simulink library "sixDoFDynamics_cl"  (R2020a)
settings: Solver=VariableStepAuto  StartTime=0.0  StopTime=10.0  RelTol=1e-3
undefined symbols (not defined in the file): init_B_vKite, init_Euler, init_OwB, init_rKite, invJKite, jKite, mKite
libraries: vrlib x2, sharedutil x1, makeOcB_cl x1
settings Model: Creator=Ayaz  LastModifiedBy=Ayaz

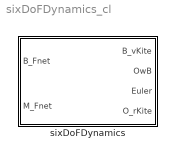
== system sixDoFDynamics_cl ==
  sixDoFDynamics : Subsystem

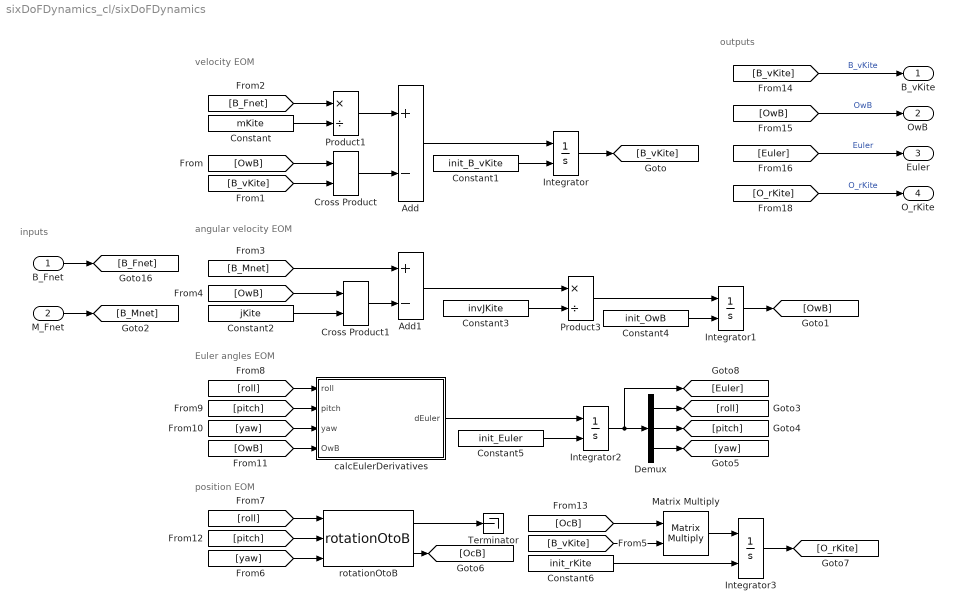
== system sixDoFDynamics_cl/sixDoFDynamics ==
  note: outputs
  note: inputs
  note: position EOM
  note: Euler angles EOM
  note: angular velocity EOM
  note: velocity EOM
  B_Fnet : Inport
  M_Fnet : Inport  Port=2
  Add : Sum  Inputs=+-
  Add1 : Sum  Inputs=+-
  Constant : Constant  Value=mKite
  Constant1 : Constant  Value=init_B_vKite
  Constant2 : Constant  Value=jKite
  Constant3 : Constant  Value=invJKite
  Constant4 : Constant  Value=init_OwB
  Constant5 : Constant  Value=init_Euler
  Constant6 : Constant  Value=init_rKite
  Cross Product : vrlib/Utilities/Cross Product
  Cross Product1 : vrlib/Utilities/Cross Product
  Demux : Demux  Outputs=3
  Integrator{,1..3} (4 alike) : Integrator  InitialConditionSource=external
  Matrix Multiply : Product  Multiplication=Matrix(*)
  Product1 : Product  Inputs=*/
  Product3 : Product  Inputs=*/
  Terminator : Terminator
  calcEulerDerivatives : Subsystem
  rotationOtoB : makeOcB_cl/rotationOtoB  SystemSampleTime=-1  Latency=0  AutoFrameSizeCalculation=off
  B_vKite : Outport
  OwB : Outport  Port=2
  Euler : Outport  Port=3
  O_rKite : Outport  Port=4
  wires:
  [OwB] -> Cross Product/1
  [B_vKite] -> Cross Product/2
  B_Fnet/1 -> [B_Fnet]
  [B_Fnet] -> Product1/1
  Constant/1 -> Product1/2
  Cross Product/1 -> Add/2
  Product1/1 -> Add/1
  Add/1 -> Integrator/1
  Constant1/1 -> Integrator/2
  Integrator/1 -> [B_vKite]
  M_Fnet/1 -> [B_Mnet]
  [OwB] -> Cross Product1/1
  Constant2/1 -> Cross Product1/2
  Cross Product1/1 -> Add1/2
  [B_Mnet] -> Add1/1
  Add1/1 -> Product3/1
  Constant3/1 -> Product3/2
  Product3/1 -> Integrator1/1
  Constant4/1 -> Integrator1/2
  Integrator1/1 -> [OwB]
  [roll] -> calcEulerDerivatives/1(roll)
  [pitch] -> calcEulerDerivatives/2(pitch)
  [yaw] -> calcEulerDerivatives/3(yaw)
  [OwB] -> calcEulerDerivatives/4(OwB)
  calcEulerDerivatives/1(dEuler) -> Integrator2/1
  Constant5/1 -> Integrator2/2
  Demux/1 -> [roll]
  Demux/2 -> [pitch]
  Demux/3 -> [yaw]
  Integrator2/1 -> [Euler], Demux/1
  [pitch] -> rotationOtoB/2
  [roll] -> rotationOtoB/1
  [yaw] -> rotationOtoB/3
  rotationOtoB/2 -> [OcB]
  [B_vKite] -> Matrix Multiply/2
  [OcB] -> Matrix Multiply/1
  rotationOtoB/1 -> Terminator/1
  Matrix Multiply/1 -> Integrator3/1
  Constant6/1 -> Integrator3/2
  Integrator3/1 -> [O_rKite]
  [B_vKite] -> B_vKite/1  "B_vKite"
  [OwB] -> OwB/1  "OwB"
  [Euler] -> Euler/1  "Euler"
  [O_rKite] -> O_rKite/1  "O_rKite"

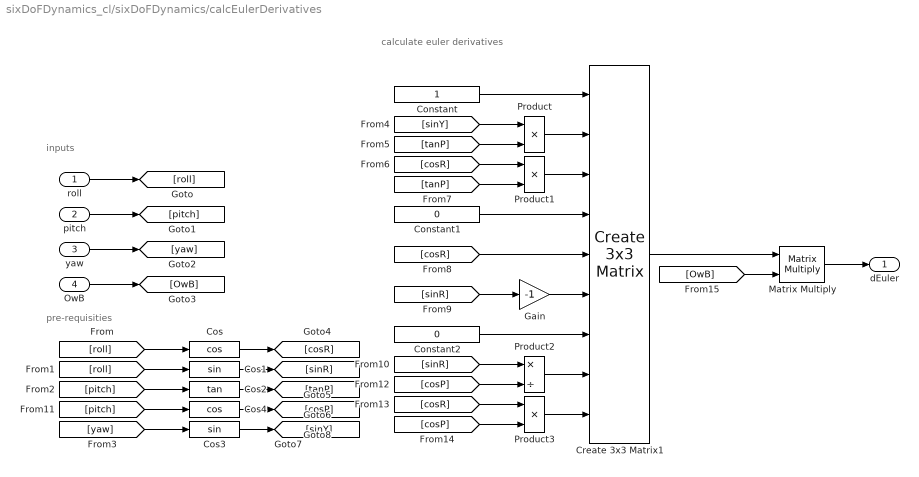
== system sixDoFDynamics_cl/sixDoFDynamics/calcEulerDerivatives ==
  note: calculate euler derivatives
  note: pre-requisities
  note: inputs
  roll : Inport
  pitch : Inport  Port=2
  yaw : Inport  Port=3
  OwB : Inport  Port=4
  Constant : Constant
  Constant1 : Constant  Value=0
  Constant2 : Constant  Value=0
  Cos : Trigonometry  Operator=cos
  Cos1 : Trigonometry
  Cos2 : Trigonometry  Operator=tan
  Cos3 : Trigonometry
  Cos4 : Trigonometry  Operator=cos
  Create 3x3 Matrix1 : sharedutil/Create 3x3 Matrix  aMode=aMode
      settings: SourceProductBaseCode=AE,PW,MT,VE,VP
  Gain : Gain  Gain=-1
  Matrix Multiply : Product  Multiplication=Matrix(*)
  Product : Product
  Product1 : Product
  Product2 : Product  Inputs=*/
  Product3 : Product
  dEuler : Outport
  wires:
  roll/1 -> [roll]
  pitch/1 -> [pitch]
  yaw/1 -> [yaw]
  OwB/1 -> [OwB]
  [roll] -> Cos/1
  [roll] -> Cos1/1
  [pitch] -> Cos2/1
  [yaw] -> Cos3/1
  Cos/1 -> [cosR]
  Cos1/1 -> [sinR]
  Cos2/1 -> [tanP]
  Cos3/1 -> [sinY]
  Constant/1 -> Create 3x3 Matrix1/1
  Product/1 -> Create 3x3 Matrix1/2
  [sinY] -> Product/1
  [tanP] -> Product/2
  Product1/1 -> Create 3x3 Matrix1/3
  [cosR] -> Product1/1
  [tanP] -> Product1/2
  Constant1/1 -> Create 3x3 Matrix1/4
  [cosR] -> Create 3x3 Matrix1/5
  [sinR] -> Gain/1
  Gain/1 -> Create 3x3 Matrix1/6
  Constant2/1 -> Create 3x3 Matrix1/7
  Product3/1 -> Create 3x3 Matrix1/9
  Product2/1 -> Create 3x3 Matrix1/8
  [sinR] -> Product2/1
  Cos4/1 -> [cosP]
  [pitch] -> Cos4/1
  [cosP] -> Product2/2
  [cosR] -> Product3/1
  [cosP] -> Product3/2
  Create 3x3 Matrix1/1 -> Matrix Multiply/1
  [OwB] -> Matrix Multiply/2
  Matrix Multiply/1 -> dEuler/1
